simulink model "Assignment3_192184_Jorge_Montalvo"  (R2019b)
settings: Solver=ode23t  StartTime=0.0  StopTime=10  MaxStep=0.1  RelTol=1e-3
libraries: powerlib x17, powerlib_meascontrol x6
settings Model: Creator=matm  LastModifiedBy=jorge
settings SolverCC: ShapePreserveControl=EnableAll  SolverResetMethod=Robust
settings DataIOCC: ReturnWorkspaceOutputs=off
settings DebuggingCC: UnconnectedInputMsg=none  UnconnectedOutputMsg=none  UnconnectedLineMsg=none  ArithmeticOperatorsInVariantConditions=warning
settings SFSimCC: SimUseLocalCustomCode=off  CustomCodeUndefinedFunction=UseInterfaceOnly
settings RTWCC: RTWUseLocalCustomCode=off
settings CodeAppCC: StateflowObjectComments=on
settings SimscapeCC: SimscapeNormalizeSystem=off

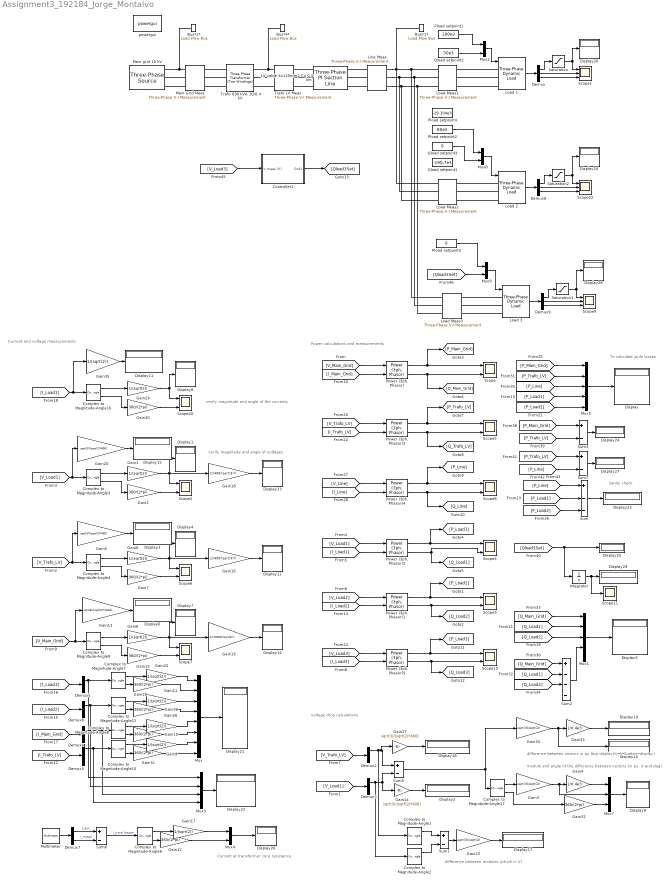
== system Assignment3_192184_Jorge_Montalvo ==
  note: verify magnitude and angle of voltages
  note: voltage drop calculations
  note: module and angle of the difference between vectors (in pu, V and deg)
  note: Current and voltage measurements
  note: difference between vectors in pu (top display) in V (bottom display)
  note: Power calculations and measurements
  note: difference between modules (ph-ph in V)
  note: verify magnitude and angle of the currents
  note: Current at transformer core resistance
  note: Sanity check
  note: To calculate joule losses
  Bus*1* : powerlib/Measurements/Load Flow Bus  LConnTagsString=a  Phases=single  Connectors=on one side  ID=Load  Vbase=400  Vref=1  Vangle=0  VLF=0.8805  VLFb=1  VLFc=1  angleLF=-1.738  angleLFb=0  angleLFc=0
      settings: SourceProductName=Simscape Electrical
  Bus*2* : powerlib/Measurements/Load Flow Bus  LConnTagsString=a  Phases=single  Connectors=on one side  ID=Slack  Vbase=10000  Vref=1  Vangle=0  VLF=1  VLFb=1  VLFc=1  angleLF=0  angleLFb=0  angleLFc=0
      settings: SourceProductName=Simscape Electrical
  Bus*4* : powerlib/Measurements/Load Flow Bus  LConnTagsString=a  Phases=single  Connectors=on one side  ID=Trafo LV  Vbase=400  Vref=1  Vangle=0  VLF=0.9929  VLFb=1  VLFc=1  angleLF=-0.6678  angleLFb=0  angleLFc=0
      settings: SourceProductName=Simscape Electrical
  Complex to Magnitude-Angle{1..4,6..10,12,16..17} (12 alike) : ComplexToMagnitudeAngle
  Controller2 : Subsystem
  Demux{,1..6,8..9} (9 alike) : Demux  Outputs=3
  Demux7 : Demux  Outputs=2
  Display{,1..29} (30 alike) : Display
      Display12 settings: Decimation=4
      Display27 settings: Format=short_e
  Gain{1,6,8..9,11,17,25..26,29,35} (10 alike) : Gain  Gain=1/(sqrt(2))
  Gain{2,7,10,12,15,28,30..32,36} (10 alike) : Gain  Gain=360/(2*pi)
  Gain13 : Gain  Gain=sqrt(3)/(sqrt(2)*10e3)
  Gain{5,14,20,27} (4 alike) : Gain  Gain=sqrt(3)/(sqrt(2)*400)
  Gain16 : Gain  Gain=1/(400/(sqrt(3)))
  Gain18 : Gain  Gain=1/(400/(sqrt(3)))
  Gain19 : Gain  Gain=1/(10000/(sqrt(3)))
  Gain23 : Gain  Gain=sqrt(3)/sqrt(2)
  Gain3 : Gain  Gain=sqrt(3)/sqrt(2)
  Gain33 : Gain  Gain=1/0.4e3
  Gain34 : Gain  Gain=sqrt(3)/sqrt(2)
  Gain4 : Gain  Gain=1/0.4e3
  Integrator : Integrator
  LV cable 4x120mm2 Cu 0.5 km : powerlib/Elements/Three-Phase PI Section Line  LConnTagsString=a|b|c  RConnTagsString=A|B|C  Frequency=50  Resistances=[ 0.1556 0.6224]  Inductances=[ 0.23e-3 0.9172e-3]  Capacitances=[920e-09 485e-09]  Length=0.5
      settings: SourceProductName=Simscape Electrical
  Line Meas : powerlib/Measurements/Three-Phase V-I Measurement  VoltageMeasurement=phase-to-ground  SetLabelV=on  LabelV=V_Line  Vpu=off  VpuLL=off  CurrentMeasurement=yes  SetLabelI=on  LabelI=I_Line  Ipu=off  Pbase=100e6  Vbase=500e3  OutputType=Complex  PhasorSimulation=on  PSBequivalent=0
      settings: SourceProductName=Simscape Electrical
  Load 1 : powerlib/Elements/Three-Phase Dynamic Load  NominalVoltage=[ 0.4e3 50 ]  ActiveReactivePowers=[100000 50000]  PositiveSequence=[0.880511 -1.73846]  ExternalControl=on  NpNq=[1 1]  TimeConstants="[0  0  0  0]"  MinimumVoltage=0.7  Tfilter=1e-4  LoadFlowParameters=[4 100000 0 0 100000]
      settings: SourceProductName=Simscape Electrical  SourceProductBaseCode=PS
  Load 2 : powerlib/Elements/Three-Phase Dynamic Load  NominalVoltage=[ 0.4e3 50 ]  ActiveReactivePowers=[80000 0]  PositiveSequence=[0.880511 -1.73846]  ExternalControl=on  NpNq=[0 0]  TimeConstants="[0  0  0  0]"  MinimumVoltage=0.7  Tfilter=1e-4  LoadFlowParameters=[4 100000 0 0 100000]
      settings: SourceProductName=Simscape Electrical  SourceProductBaseCode=PS
  Load 3 : powerlib/Elements/Three-Phase Dynamic Load  NominalVoltage=[ 0.4e3 50 ]  ActiveReactivePowers=[0 0]  PositiveSequence=[0.880511 -1.73846]  ExternalControl=on  NpNq=[0 0]  TimeConstants="[0  0  0  0]"  MinimumVoltage=0.7  Tfilter=1e-4  LoadFlowParameters=[4 100000 0 0 100000]
      settings: SourceProductName=Simscape Electrical  SourceProductBaseCode=PS
  Load Meas1 : powerlib/Measurements/Three-Phase V-I Measurement  VoltageMeasurement=phase-to-ground  SetLabelV=on  LabelV=V_Load1  Vpu=off  VpuLL=off  CurrentMeasurement=yes  SetLabelI=on  LabelI=I_Load1  Ipu=off  Pbase=100e6  Vbase=500e3  OutputType=Complex  PhasorSimulation=on  PSBequivalent=0
      settings: SourceProductName=Simscape Electrical
  Load Meas2 : powerlib/Measurements/Three-Phase V-I Measurement  VoltageMeasurement=phase-to-ground  SetLabelV=on  LabelV=V_Load2  Vpu=off  VpuLL=off  CurrentMeasurement=yes  SetLabelI=on  LabelI=I_Load2  Ipu=off  Pbase=100e6  Vbase=500e3  OutputType=Complex  PhasorSimulation=on  PSBequivalent=0
      settings: SourceProductName=Simscape Electrical
  Load Meas3 : powerlib/Measurements/Three-Phase V-I Measurement  VoltageMeasurement=phase-to-ground  SetLabelV=on  LabelV=V_Load3  Vpu=off  VpuLL=off  CurrentMeasurement=yes  SetLabelI=on  LabelI=I_Load3  Ipu=off  Pbase=100e6  Vbase=500e3  OutputType=Complex  PhasorSimulation=on  PSBequivalent=0
      settings: SourceProductName=Simscape Electrical
  Main Grid Meas : powerlib/Measurements/Three-Phase V-I Measurement  VoltageMeasurement=phase-to-ground  SetLabelV=on  LabelV=V_Main_Grid  Vpu=off  VpuLL=off  CurrentMeasurement=yes  SetLabelI=on  LabelI=I_Main_Grid  Ipu=off  Pbase=100e6  Vbase=500e3  OutputType=Complex  PhasorSimulation=on  PSBequivalent=0
      settings: SourceProductName=Simscape Electrical
  Main grid 10 kV : powerlib/Electrical Sources/Three-Phase Source  InternalConnection=Yg  VoltagePhases=off  Voltage=(10000)*1.0017  PhaseAngle=0.22586  Voltage_phases=[25e3 25e3 25e3]/sqrt(3)  PhaseAngles_phases=[0 -120 +120]  Frequency=50  NonIdealSource=on  SpecifyImpedance=on  Resistance=0.8929  Inductance=16.58e-3  ShortCircuitLevel=50e6  BaseVoltage=10e3  XRratio=10  BusType=swing  Pref=10e3  Qref=0  Prefabc=[10e3, 10e3, 10e3]  Qrefabc=[0, 0, 0]  Qmin=-inf  Qmax=inf
      settings: SourceProductName=Simscape Electrical
  Multimeter : powerlib/Measurements/Multimeter  PhasorSimulation=on  OutputType=Complex  sel=[13 16]  L=21  Gain=[1 1]  yselected={'Iexc_A: Trafo 630 kVA 10//0.4 kV','Imag_A: Trafo 630 kVA 10//0.4 kV'};  PSBOutputType=1  PSBequivalent=0  AxesSetting=[0,0.1,-100,100]  Display=0  SavedBlockNames=-11
      settings: SourceProductName=Simscape Electrical
  Mux : Mux  Inputs=8
  Mux1 : Mux  Inputs=5
  Mux{2,4,8..9} (4 alike) : Mux  Inputs=2
  Mux3 : Mux
  Mux5 : Mux  Inputs=5
  Mux7 : Mux  Inputs=3
  Pload setpoint1 : Constant  Value=100e3
  Pload setpoint2 : Constant  Value=80e3
  Pload setpoint3 : Constant  Value=0
  Pload setpoint4 : Constant  Value=-29.104e3
  Power (3ph, Phasor){,1..5} (6 alike) : powerlib_meascontrol/Measurements/Power (3ph, Phasor)
      settings: SourceProductName=Simscape Electrical  SourceProductBaseCode=PS
  Qload setpoint1 : Constant  Value=-190.7e3
  Qload setpoint2 : Constant  Value=50e3
  Qload setpoint3 : Constant  Value=0
  Saturation : Saturate  UpperLimit=1.15  LowerLimit=0.85
  Saturation1 : Saturate  UpperLimit=1.15  LowerLimit=0.85
  Saturation2 : Saturate  UpperLimit=1.15  LowerLimit=0.85
  Scope{,2..8,10,20} (10 alike) : Scope  NumInputPorts=2
  Scope1 : Scope  NumInputPorts=3
  Scope11 : Scope
  Scope22 : Scope  NumInputPorts=3
  Scope9 : Scope  NumInputPorts=3
  Sum : Sum  Inputs=+--
  Sum{1,3,5..7} (5 alike) : Sum  Inputs=+-
  Sum2 : Sum  Inputs=+---
  Trafo 630 kVA 10/0.4 kV : powerlib/Elements/Three-Phase Transformer (Two Windings)  Winding1Connection=Yg  Winding2Connection=Yg  CoreType=Three single-phase transformers  SetSaturation=off  Hysteresis=off  DataFile='hysteresis'  SetInitialFlux=off  Measurements=All measurements (V I Fluxes)  UNITS=pu  NominalPower=[ 630e3 , 50 ]  Winding1=[10000 0.005 0.0195]  Winding2=[400 0.005 0.0195]  Rm=500  Lm=500  L0=0.5  Saturation=[0 0;0.0024 1.2;1 1.52]  InitialFluxes=[0.8 -0.8 0.7]  BreakLoop=off  DiscreteSolver=Trapezoidal iterative  DataType=off  TransfoNumber=1
      settings: SourceProductName=Simscape Electrical
  Trafo LV Meas : powerlib/Measurements/Three-Phase V-I Measurement  VoltageMeasurement=phase-to-ground  SetLabelV=on  LabelV=V_Trafo_LV  Vpu=off  VpuLL=off  CurrentMeasurement=yes  SetLabelI=on  LabelI=I_Trafo_LV  Ipu=off  Pbase=100e6  Vbase=500e3  OutputType=Complex  PhasorSimulation=on  PSBequivalent=0
      settings: SourceProductName=Simscape Electrical
  powergui : powerlib/powergui  Priority=1  SimulationMode=Phasor  SampleTime=50e-6  frequency=50  Iterations=50  frequencyindice=50  Pbase=1e6  ErrMax=0.0001  UnitsV=kV  UnitsW=kW  buscounter=7  FunctionMessages=off  echomessages=off  EnableUseOfTLC=off  CurrentSourceSwitches=off  DisableSnubberDevices=off  DisableRonSwitches=off  DisableVfSwitches=off  DisplayEquations=off  AutomaticDiscreteSolvers=off  SolverType=Tustin/Backward Euler (TBE)  Interpol=off  ExternalGateDelay=off  methode=off  Ts=10  x0status=blocks  SPID=off  SwTol=0  HookPort=off  NonlinearTolerance=1e-4  nMaxIteration=100  ContinueOnMaxIteration=off  RestoreLinks=warning  ResistiveCurrentMeasurement=off  Frange=[0:2:500]  Ylog=off  Xlog=on  ShowGrid=off  save=off  variable=ZData  structure=ScopeData  ZoomFFT=off  StartTime=0.0  cycles=1  DisplayStyle=1  fundamental=60  FreqAxis=off  MaxFrequency=1000  frequencyindicesteady=1  RmsSteady=2  display=off
      settings: SourceProductName=Simscape Electrical
  wires:
  Load 1/1 -> Demux/1
  Demux/3 -> Scope1/3
  Demux/2 -> Scope1/2
  Demux/1 -> Saturation/1
  Saturation/1 -> Display20/1, Scope1/1
  Mux8/1 -> Load 2/1
  Load 2/1 -> Demux6/1
  Demux6/3 -> Scope22/3
  Demux6/2 -> Scope22/2
  Demux6/1 -> Saturation2/1
  Saturation2/1 -> Display16/1, Scope22/1
  Complex to Magnitude-Angle17/2 -> Gain32/1
  Gain30/1 -> Scope20/2
  Complex to Magnitude-Angle4/2 -> Gain7/1
  Gain7/1 -> Scope6/2
  Gain2/1 -> Scope2/2
  Gain1/1 -> Scope2/1, Gain18/1, Display1/1
  Complex to Magnitude-Angle16/1 -> Gain29/1
  Gain29/1 -> Scope20/1, Display8/1
  [I_Main_Grid] -> "Power (3ph, Phasor)"/2
  Complex to Magnitude-Angle16/2 -> Gain30/1
  [I_Load1] -> "Power (3ph, Phasor)2"/2
  [V_Load1] -> "Power (3ph, Phasor)2"/1
  Gain19/1 -> Display14/1
  Gain13/1 -> Display6/1
  [I_Load1] -> Gain35/1, Complex to Magnitude-Angle16/1
  "Power (3ph, Phasor)2"/2 -> [Q_Load1], Scope4/2
  "Power (3ph, Phasor)"/1 -> Scope/1, [P_Main_Grid]
  Gain8/1 -> Scope7/1, Gain19/1, Display7/1
  Gain16/1 -> Display12/1
  Gain15/1 -> Scope7/2
  [V_Load1] -> Demux3/1
  Gain14/1 -> Display2/1
  Complex to Magnitude-Angle17/1 -> Gain3/1
  Complex to Magnitude-Angle3/1 -> Gain1/1
  Complex to Magnitude-Angle4/1 -> Gain6/1
  Gain6/1 -> Gain16/1, Scope6/1, Display4/1
  [V_Load1] -> Complex to Magnitude-Angle3/1, Gain20/1
  "Power (3ph, Phasor)"/2 -> Scope/2, [Q_Main_Grid]
  Sum5/1 -> Complex to Magnitude-Angle17/1, Gain34/1
  [V_Trafo_LV] -> Demux2/1
  Gain34/1 -> Gain33/1, Display10/1
  Complex to Magnitude-Angle9/1 -> Gain8/1
  Demux3/1 -> Gain14/1, Sum5/2, Complex to Magnitude-Angle2/1
  [V_Main_Grid] -> "Power (3ph, Phasor)"/1
  Mux7/1 -> Display9/1
  "Power (3ph, Phasor)2"/1 -> [P_Load1], Scope4/1
  Demux2/1 -> Sum5/1, Gain27/1, Complex to Magnitude-Angle1/1
  Gain35/1 -> Display11/1
  Gain27/1 -> Display18/1
  [V_Main_Grid] -> Gain13/1, Complex to Magnitude-Angle9/1
  Complex to Magnitude-Angle3/2 -> Gain2/1
  Complex to Magnitude-Angle1/1 -> Sum1/1
  Gain32/1 -> Mux7/3
  Gain20/1 -> Display15/1
  Gain18/1 -> Display13/1
  Complex to Magnitude-Angle9/2 -> Gain15/1
  Gain3/1 -> Mux7/2, Gain4/1
  Sum1/1 -> Gain23/1
  Gain33/1 -> Display19/1
  [V_Trafo_LV] -> Complex to Magnitude-Angle4/1, Gain5/1
  Gain4/1 -> Mux7/1
  Gain23/1 -> Display17/1
  Complex to Magnitude-Angle2/1 -> Sum1/2
  Gain5/1 -> Display3/1
  "Power (3ph, Phasor)1"/1 -> Scope3/1, [P_Load2]
  "Power (3ph, Phasor)1"/2 -> Scope3/2, [Q_Load2]
  [V_Load2] -> "Power (3ph, Phasor)1"/1
  [I_Load2] -> "Power (3ph, Phasor)1"/2
  [P_Main_Grid] -> Mux5/1
  [P_Load2] -> Mux5/5
  [P_Load1] -> Mux5/4
  [P_Line] -> Sum/1
  Mux5/1 -> Display/1
  Sum/1 -> Display23/1
  Mux1/1 -> Display5/1
  [Q_Load1] -> Mux1/2
  [Q_Main_Grid] -> Mux1/1
  [Q_Main_Grid] -> Sum2/1
  [Q_Load2] -> Mux1/3
  [Q_Load2] -> Sum2/3
  [Q_Load1] -> Sum2/2
  Sum2/1 -> Mux1/4
  Pload setpoint1/1 -> Mux2/1
  Mux2/1 -> Load 1/1
  Qload setpoint2/1 -> Mux2/2
  Complex to Magnitude-Angle10/2 -> Gain31/1
  Gain11/1 -> Mux/3
  Gain25/1 -> Mux/1
  Gain36/1 -> Mux/4
  Mux3/1 -> Display22/1
  Gain10/1 -> Mux/6
  Complex to Magnitude-Angle8/1 -> Gain26/1
  [I_Load1] -> Demux1/1
  Complex to Magnitude-Angle8/2 -> Gain10/1
  Demux4/1 -> Mux3/3, Complex to Magnitude-Angle8/1
  Gain31/1 -> Mux/8
  Gain9/1 -> Mux/7
  Gain26/1 -> Mux/5
  Demux1/1 -> Mux3/1, Complex to Magnitude-Angle7/1
  Gain28/1 -> Mux/2
  Demux8/1 -> Mux3/2, Complex to Magnitude-Angle12/1
  [I_Load2] -> Demux8/1
  Complex to Magnitude-Angle7/1 -> Gain25/1
  Complex to Magnitude-Angle12/2 -> Gain36/1
  [I_Trafo_LV] -> Demux5/1
  Complex to Magnitude-Angle7/2 -> Gain28/1
  Mux/1 -> Display21/1
  Complex to Magnitude-Angle12/1 -> Gain11/1
  Complex to Magnitude-Angle10/1 -> Gain9/1
  [I_Main_Grid] -> Demux4/1
  [I_Trafo_LV] -> "Power (3ph, Phasor)3"/2
  "Power (3ph, Phasor)3"/2 -> Scope5/2, [Q_Trafo_LV]
  [V_Trafo_LV] -> "Power (3ph, Phasor)3"/1
  "Power (3ph, Phasor)3"/1 -> Scope5/1, [P_Trafo_LV]
  "Power (3ph, Phasor)4"/1 -> Scope8/1, [P_Line]
  "Power (3ph, Phasor)4"/2 -> Scope8/2, [Q_Line]
  [I_Line] -> "Power (3ph, Phasor)4"/2
  [V_Line] -> "Power (3ph, Phasor)4"/1
  [P_Trafo_LV] -> Mux5/2
  [P_Line] -> Mux5/3
  [P_Trafo_LV] -> Sum3/2
  [P_Main_Grid] -> Sum3/1
  Sum3/1 -> Display24/1
  Demux5/1 -> Mux3/4, Complex to Magnitude-Angle10/1
  Multimeter/1 -> Demux7/1
  Gain12/1 -> Mux4/2
  Complex to Magnitude-Angle6/2 -> Gain12/1
  Gain17/1 -> Mux4/1
  Complex to Magnitude-Angle6/1 -> Gain17/1
  Mux4/1 -> Display26/1
  Demux7/1 -> Sum6/1  "I_exc"
  Demux7/2 -> Sum6/2  "I_magn"
  Sum6/1 -> Complex to Magnitude-Angle6/1  "I_core losses"
  Sum7/1 -> Display27/1
  [P_Line] -> Sum7/2
  [P_Trafo_LV] -> Sum7/1
  [P_Load1] -> Sum/2
  [P_Load2] -> Sum/3
  [Qload3Set] -> Display25/1, Integrator/1
  Controller2/1(Out1) -> [Qload3Set]
  [V_Load3] -> Controller2/1(V meas (V))
  Demux9/3 -> Scope9/3
  Demux9/2 -> Scope9/2
  Mux9/1 -> Load 3/1
  Saturation1/1 -> Display28/1, Scope9/1
  Demux9/1 -> Saturation1/1
  Load 3/1 -> Demux9/1
  Pload setpoint3/1 -> Mux9/1
  [Qload3Set] -> Mux9/2
  Qload setpoint3/1 -> Mux8/2
  Pload setpoint2/1 -> Mux8/1
  [I_Load3] -> "Power (3ph, Phasor)5"/2
  "Power (3ph, Phasor)5"/2 -> Scope10/2, [Q_Load3]
  [V_Load3] -> "Power (3ph, Phasor)5"/1
  "Power (3ph, Phasor)5"/1 -> Scope10/1, [P_Load3]
  Integrator/1 -> Scope11/1, Display29/1
  connections:
  Main grid 10 kV/RConn1 -- Main Grid Meas/LConn1 -- Bus*2*/LConn1
  Main Grid Meas/LConn2 -- Main grid 10 kV/RConn2
  Main Grid Meas/LConn3 -- Main grid 10 kV/RConn3
  Trafo 630 kVA 10/0.4 kV/LConn3 -- Main Grid Meas/RConn3
  Trafo 630 kVA 10/0.4 kV/LConn1 -- Main Grid Meas/RConn1
  Trafo 630 kVA 10/0.4 kV/LConn2 -- Main Grid Meas/RConn2
  Trafo 630 kVA 10/0.4 kV/RConn1 -- Trafo LV Meas/LConn1 -- Bus*4*/LConn1
  Trafo LV Meas/LConn2 -- Trafo 630 kVA 10/0.4 kV/RConn2
  Trafo LV Meas/LConn3 -- Trafo 630 kVA 10/0.4 kV/RConn3
  LV cable 4x120mm2 Cu 0.5 km/LConn1 -- Trafo LV Meas/RConn1
  Trafo LV Meas/RConn2 -- LV cable 4x120mm2 Cu 0.5 km/LConn2
  LV cable 4x120mm2 Cu 0.5 km/LConn3 -- Trafo LV Meas/RConn3
  Load Meas2/LConn1 -- Load Meas1/LConn1 -- Load Meas3/LConn1 -- Line Meas/RConn1 -- Bus*1*/LConn1
  Load Meas2/LConn2 -- Load Meas1/LConn2 -- Load Meas3/LConn2 -- Line Meas/RConn2
  Load Meas2/LConn3 -- Load Meas3/LConn3 -- Load Meas1/LConn3 -- Line Meas/RConn3
  Load 1/LConn3 -- Load Meas1/RConn3
  Load 1/LConn2 -- Load Meas1/RConn2
  Load 1/LConn1 -- Load Meas1/RConn1
  Load 2/LConn1 -- Load Meas2/RConn1
  Load 2/LConn2 -- Load Meas2/RConn2
  Load 2/LConn3 -- Load Meas2/RConn3
  Line Meas/LConn1 -- LV cable 4x120mm2 Cu 0.5 km/RConn1
  Line Meas/LConn2 -- LV cable 4x120mm2 Cu 0.5 km/RConn2
  Line Meas/LConn3 -- LV cable 4x120mm2 Cu 0.5 km/RConn3
  Load 3/LConn2 -- Load Meas3/RConn2
  Load 3/LConn3 -- Load Meas3/RConn3
  Load 3/LConn1 -- Load Meas3/RConn1

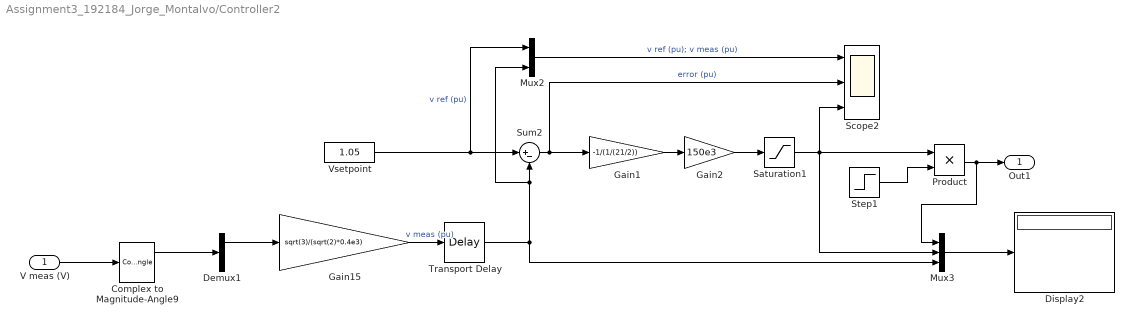
== system Assignment3_192184_Jorge_Montalvo/Controller2 ==
  V meas (V) : Inport
  Complex to Magnitude-Angle9 : ComplexToMagnitudeAngle
  Demux1 : Demux  Outputs=3
  Display2 : Display
  Gain1 : Gain  Gain=-1/(1/(21/2))
  Gain15 : Gain  Gain=sqrt(3)/(sqrt(2)*0.4e3)
  Gain2 : Gain  Gain=150e3
  Mux2 : Mux  Inputs=2
  Mux3 : Mux  Inputs=3
  Product : Product
  Saturation1 : Saturate  UpperLimit=150e3  LowerLimit=-150e3
  Scope2 : Scope  NumInputPorts=3
  Step1 : Step  Time=3  SampleTime=0
  Sum2 : Sum  Inputs=|+-
  Transport Delay : TransportDelay  DelayTime=0.5
  Vsetpoint : Constant  Value=1.05
  Out1 : Outport  VectorParamsAs1DForOutWhenUnconnected=off
  wires:
  Product/1 -> Mux3/1, Out1/1
  Demux1/1 -> Gain15/1
  Sum2/1 -> Scope2/2, Gain1/1  "error (pu)"
  Complex to Magnitude-Angle9/1 -> Demux1/1
  Vsetpoint/1 -> Mux2/1, Sum2/1  "v ref (pu)"
  Gain15/1 -> Transport Delay/1  "v meas (pu)"
  Step1/1 -> Product/2
  Gain1/1 -> Gain2/1
  V meas (V)/1 -> Complex to Magnitude-Angle9/1
  Mux2/1 -> Scope2/1  "v ref (pu); v meas (pu)"
  Gain2/1 -> Saturation1/1
  Mux3/1 -> Display2/1
  Saturation1/1 -> Mux3/2, Product/1, Scope2/3
  Transport Delay/1 -> Mux3/3, Mux2/2, Sum2/2
